simulink model "soc_dvbs2_fpga"  (R2025b)
settings: Solver=FixedStepDiscrete  StartTime=0.0  StopTime=0  RelTol=1e-3
InitFcn:
  | soc_dvbs2_init;
values from neighbouring files (symbols this model uses):
  Rsym = 4e6    (= 4000000)    [soc_dvbs2_init.m]
  soc_dvbs2_txPacketBits = [1 1 0 1 0 1 1 1 0 1 1 1 ... (2972 elements, 2972x1)]    [soc_dvbs2_txPacketBits.mat]
  syncWord = (dec2bin(hex2dec('AC')) - '0').'    [soc_dvbs2_init.m]
  txDataOut = txobj(frameBits(:))    [soc_dvbs2_init.m]
  txFiltCoeff = txobj.pTxFilterCoeff    [soc_dvbs2_init.m]
undefined symbols (not defined in the file or in its folder): Add, coefficientsLog, coefficientsSqrt1, coefficientsSqrt2, dataBits, designMultirateFIR, noisePow, NumBits1, NumBits2, seedsURNG1, seedsURNG2, Shift, Slope1, Slope2, soc_dvbs2_designFIRFilter, txDataOutS1, txDataOutS10, txDataOutS12, txDataOutS13, txDataOutS14, txDataOutS15, txDataOutS16, txDataOutS18, txDataOutS19, txDataOutS2, txDataOutS20, txDataOutS21, txDataOutS22, txDataOutS24, txDataOutS25, txDataOutS26, txDataOutS27, txDataOutS3, txDataOutS4, txDataOutS5, txDataOutS6, txDataOutS7, txDataOutS8, txDataOutS9
libraries: simulink x214, hdlsllib x211, dspsigops x22, dsphdlfiltering2 x8, dsphdlsigops2 x5, commseqgen3 x5, dsphdlmathfun2 x3, hwlogicconnlib x2, whdledac x2, commhdlcrc x2, whdlutilities x1, whdlmod x1
(part 7 of 12)

== system soc_dvbs2_fpga/DVBS2/DVBS2 TxRx/DVB-S2 HDL Receiver/Synchronizer and PL Header Decoder/Time Frequency and Coarse Phase Synchronizer/Coarse Phase Synchronizer/Coarse Phase Estimator ==
  dataIn : Inport
  pilotIdx : Inport  Port=2
  pilotValid : Inport  Port=3
  Add3 : Sum  Inputs=++|  OutDataTypeStr=Inherit: Inherit via back propagation
  Compare To Constant1 : simulink/Logic and Bit Operations/Compare To Constant  relop===  const=config.PilotMaxIdx  OutDataTypeStr=boolean
  Compare To Constant2 : simulink/Logic and Bit Operations/Compare To Constant  relop===  const=config.PilotMinIdx  OutDataTypeStr=boolean
  Data Type Duplicate : DataTypeDuplicate
  Data Type Conversion : DataTypeConversion  OutDataTypeStr=fixdt(1,17,14)  SaturateOnIntegerOverflow=off  RndMeth=Floor
  Delay{,1,15..17} (5 alike) : Delay  DelayLength=1
  Delay{8..11} (4 alike) : Delay  DelayLength=1  InitialCondition=0
  Delay{2..7,12..14,20} (10 alike) : Delay  InitialCondition=0
  Gain : Gain  Gain=conj(config.Pilot)  OutDataTypeStr=Inherit: Same as input
      mask init:
      | Simulink.suppressDiagnostic(gcb, 'SimulinkFixedPoint:util:fxpParameterPrecisionLoss');
  Gain1 : Gain  Gain=1/32  ParamDataTypeStr=fixdt(0,5,5)  OutDataTypeStr=Inherit: Same as input
  Logical Operator : Logic  AllPortsSameDT=off  OutDataTypeStr=boolean
  Logical Operator1 : Logic  AllPortsSameDT=off  OutDataTypeStr=boolean
  Unit Delay Enabled Resettable Synchronous : hdlsllib/Discrete/Unit Delay Enabled Resettable Synchronous  InitialCondition=0.0  SampleTime=-1
  estimate : Outport
  estValid : Outport  Port=2
  wires:
  Delay17/1 -> estValid/1
  Delay16/1 -> Delay13/1
  Delay15/1 -> Compare To Constant1/1
  pilotValid/1 -> Delay16/1, Delay5/1, Delay/1
  Logical Operator1/1 -> Delay12/1
  Compare To Constant1/1 -> Delay14/1
  Delay13/1 -> Logical Operator1/2
  Delay14/1 -> Logical Operator1/1
  Delay12/1 -> Delay11/1
  Delay11/1 -> Delay17/1
  Data Type Conversion/1 -> Delay8/1
  Delay10/1 -> Unit Delay Enabled Resettable Synchronous/3
  Delay9/1 -> Unit Delay Enabled Resettable Synchronous/2
  Delay8/1 -> Add3/2, Data Type Duplicate/1
  Gain1/1 -> Data Type Conversion/1
  Delay3/1 -> Delay9/1
  Delay2/1 -> Gain1/1
  Add3/1 -> Unit Delay Enabled Resettable Synchronous/1, Data Type Duplicate/2
  Delay20/1 -> Delay10/1
  Unit Delay Enabled Resettable Synchronous/1 -> Add3/1, estimate/1
  Delay7/1 -> Delay3/1
  Delay6/1 -> Logical Operator/1
  Delay5/1 -> Logical Operator/2
  Delay4/1 -> Gain/1
  Compare To Constant2/1 -> Delay6/1
  Logical Operator/1 -> Delay20/1
  Delay1/1 -> Delay4/1
  Gain/1 -> Delay2/1
  pilotIdx/1 -> Delay15/1, Compare To Constant2/1
  Delay/1 -> Delay7/1
  dataIn/1 -> Delay1/1

== system soc_dvbs2_fpga/DVBS2/DVBS2 TxRx/DVB-S2 HDL Receiver/Synchronizer and PL Header Decoder/Time Frequency and Coarse Phase Synchronizer/Coarse Phase Synchronizer/Unwrapping algorithm ==
  note: Wrap on overflow with data type
      | signed and 1 intergral bit
      | will wrap the output to
      | lie in between -1 to 1
  u : Inport
  E : Inport  Port=2
  Add : Sum  Inputs=+-  OutDataTypeStr=Inherit: Same as first input
  Add1 : Sum  Inputs=|++  OutDataTypeStr=Inherit: Same as first input
  Complex to Magnitude-Angle HDL Optimized : dsphdlmathfun2/Complex to Magnitude-Angle  NumIterationsSource=Auto  NumIterations=10  OutputFormat=Angle  AngleFormat=Normalized  ScaleOutput=on  ScalingMethod=Shift-Add  SimulateUsing=Code generation
  Constant : Constant  Value=true  SampleTime=-1
  Data Type Conversion : DataTypeConversion  OutDataTypeStr=fixdt(1,25,20)  SaturateOnIntegerOverflow=off  RndMeth=Floor
  Data Type Conversion1 : DataTypeConversion  OutDataTypeStr=fixdt(1,21,21)  SaturateOnIntegerOverflow=off  RndMeth=Floor
  Data Type Conversion2 : DataTypeConversion  OutDataTypeStr=fixdt(1,21,0)  ConvertRealWorld=Stored Integer (SI)  SaturateOnIntegerOverflow=off  RndMeth=Floor
  Gain1 : Gain  Gain=1/2  ParamDataTypeStr=fixdt(0,1,1)
  NCO HDL Optimized : dsphdlsigops2/NCO  PhaseIncrementSource=Property  PhaseIncrement=0  PhaseOffsetSource=Input port  PhaseOffset=0  DitherSource=None  NumDitherBits=4  SamplesPerFrame=1  LUTCompress=off  ResetAction=off  Waveform=Complex exponential  PhasePort=off  SimulateUsing=Code generation  AccumulatorWL=21  PhaseQuantization=on  NumQuantizerAccumulatorBits=14  OutputDataType=Binary point scaling  OutputWL=16  OutputFL=14
  PrevEst : hdlsllib/Discrete/Unit Delay Enabled Synchronous  InitialCondition=0.0  SampleTime=-1
  Terminator : Terminator
  currentEst : hdlsllib/Discrete/Unit Delay Enabled Synchronous  InitialCondition=0.0  SampleTime=-1
  estimate : Outport  VectorParamsAs1DForOutWhenUnconnected=off
  wires:
  Add/1 -> Data Type Conversion/1
  PrevEst/1 -> Add1/2, Add/2
  NCO HDL Optimized/2 -> Terminator/1
  Constant/1 -> NCO HDL Optimized/2
  Data Type Conversion2/1 -> NCO HDL Optimized/1
  Data Type Conversion1/1 -> Data Type Conversion2/1
  Data Type Conversion/1 -> Add1/1
  Complex to Magnitude-Angle HDL Optimized/1 -> currentEst/1
  E/1 -> Complex to Magnitude-Angle HDL Optimized/2
  Gain1/1 -> Data Type Conversion1/1
  NCO HDL Optimized/1 -> estimate/1
  Add1/1 -> PrevEst/1, Gain1/1
  currentEst/1 -> Add/1
  Complex to Magnitude-Angle HDL Optimized/2 -> currentEst/2, PrevEst/2
  u/1 -> Complex to Magnitude-Angle HDL Optimized/1

== system soc_dvbs2_fpga/DVBS2/DVBS2 TxRx/DVB-S2 HDL Receiver/Synchronizer and PL Header Decoder/Time Frequency and Coarse Phase Synchronizer/Fine Frequency Synchronizer/Modified L and R Algorithm ==
  z : Inport
  zvalid : Inport  Port=2
  pilotIdx : Inport  Port=3
  Compare To Constant2 : simulink/Logic and Bit Operations/Compare To Constant  relop===  const=config.PilotMaxIdx  OutDataTypeStr=boolean
  Complex to Magnitude-Angle HDL Optimized : dsphdlmathfun2/Complex to Magnitude-Angle  NumIterationsSource=Auto  NumIterations=10  OutputFormat=Angle  AngleFormat=Normalized  ScaleOutput=on  ScalingMethod=Shift-Add  SimulateUsing=Code generation
  Data Type Conversion : DataTypeConversion  OutDataTypeStr=fixdt(1,21,21)  SaturateOnIntegerOverflow=off  RndMeth=Floor
  Data Type Conversion1 : DataTypeConversion  OutDataTypeStr=fixdt(1,43,26)  SaturateOnIntegerOverflow=off  RndMeth=Floor
  Data Type Conversion3 : DataTypeConversion  OutDataTypeStr=fixdt(1,43,40)  ConvertRealWorld=Stored Integer (SI)  SaturateOnIntegerOverflow=off  RndMeth=Floor
  Delay : Delay
  Delay1 : Delay
  Delay2 : Delay
  Delay3 : Delay  DelayLength=28
  Delay4 : Delay  DelayLength=1
  Gain : Gain  Gain=fi(1/19,0,16,16)  ParamDataTypeStr=Inherit: Inherit from 'Gain'  OutDataTypeStr=Inherit: Same as input
  L and R Algorithm 18 point : Subsystem
  Logical Operator : Logic  AllPortsSameDT=off  OutDataTypeStr=boolean
  Moving Average : Subsystem
  Terminator : Terminator
  Unit Delay Enabled Synchronous : hdlsllib/Discrete/Unit Delay Enabled Synchronous  InitialCondition=0.0  SampleTime=-1
  estOut : Outport
  wires:
  Complex to Magnitude-Angle HDL Optimized/2 -> Terminator/1, Unit Delay Enabled Synchronous/2
  Unit Delay Enabled Synchronous/1 -> Delay4/1
  Data Type Conversion1/1 -> Data Type Conversion3/1
  Moving Average/2(validOut) -> Complex to Magnitude-Angle HDL Optimized/2
  Data Type Conversion3/1 -> Complex to Magnitude-Angle HDL Optimized/1
  Complex to Magnitude-Angle HDL Optimized/1 -> Unit Delay Enabled Synchronous/1
  z/1 -> L and R Algorithm 18 point/1(z)
  Moving Average/1(dataOut) -> Data Type Conversion1/1
  Logical Operator/1 -> Delay3/1
  Compare To Constant2/1 -> Logical Operator/2
  Delay4/1 -> Delay1/1
  Delay2/1 -> Data Type Conversion/1
  Delay1/1 -> Gain/1
  Delay3/1 -> Delay/1
  Data Type Conversion/1 -> estOut/1
  Gain/1 -> Delay2/1
  zvalid/1 -> L and R Algorithm 18 point/2(zvalid), Logical Operator/1
  L and R Algorithm 18 point/1(dataIn) -> Moving Average/1(dataIn)
  Delay/1 -> Moving Average/2(validIn)
  pilotIdx/1 -> Compare To Constant2/1

== system soc_dvbs2_fpga/DVBS2/DVBS2 TxRx/DVB-S2 HDL Receiver/Synchronizer and PL Header Decoder/Time Frequency and Coarse Phase Synchronizer/Fine Gain Control/Reciprocal ==
  dataIn : Inport
  Compare To Constant : simulink/Logic and Bit Operations/Compare To Constant  relop=<  const=0  OutDataTypeStr=boolean
  Compare To Constant1 : simulink/Logic and Bit Operations/Compare To Constant  relop===  const=0  OutDataTypeStr=boolean
  Constant : Constant  OutDataTypeStr=Inherit: Inherit via back propagation  SampleTime=-1
  Data Type Duplicate : DataTypeDuplicate
  Data Type Conversion : DataTypeConversion  OutDataTypeStr=fixdt(1,WL,0)  ConvertRealWorld=Stored Integer (SI)  SaturateOnIntegerOverflow=off  RndMeth=Floor
  Data Type Conversion1 : DataTypeConversion  OutDataTypeStr=fixdt(0,LUTAddrWL,0)  ConvertRealWorld=Stored Integer (SI)  SaturateOnIntegerOverflow=off  RndMeth=Floor
      mask init:
      | Simulink.suppressDiagnostic(gcb, 'SimulinkFixedPoint:util:Overflowoccurred');
  Data Type Conversion2 : DataTypeConversion  OutDataTypeStr=fixdt(0,WL-LUTAddrWL,0)  ConvertRealWorld=Stored Integer (SI)  SaturateOnIntegerOverflow=off  RndMeth=Floor
  Delay : Delay  DelayLength=1
  Delay1 : Delay  DelayLength=1
  Delay2 : Delay  DelayLength=1
  Delay3 : Delay  DelayLength=7
  Extract Bits : simulink/Logic and Bit Operations/Extract Bits  bitsToExtract=Range ending with least significant bit  numBits=LUTAddrWL  bitIdxRange=[0 7]  outScalingMode=Treat bit field as an integer
  Function Impl : Subsystem
  Switch : Switch  Criteria=u2 > Threshold  SaturateOnIntegerOverflow=off  InputSameDT=off
  dataOut : Outport
  wires:
  Constant/1 -> Switch/1, Data Type Duplicate/1
  Compare To Constant1/1 -> Switch/2
  Delay3/1 -> Compare To Constant1/1
  Switch/1 -> dataOut/1
  Data Type Conversion2/1 -> Function Impl/1(switch)
  Delay2/1 -> Data Type Conversion1/1
  Delay1/1 -> Data Type Conversion2/1
  Delay/1 -> Extract Bits/1, Compare To Constant/1
  Function Impl/1(functionValues) -> Switch/3, Data Type Duplicate/2
  Data Type Conversion1/1 -> Function Impl/2(LUTAddr)
  Compare To Constant/1 -> Delay1/1
  Data Type Conversion/1 -> Delay/1
  Extract Bits/1 -> Delay2/1
  dataIn/1 -> Data Type Conversion/1, Delay3/1

== system soc_dvbs2_fpga/DVBS2/DVBS2 TxRx/DVB-S2 HDL Receiver/Synchronizer and PL Header Decoder/Time Frequency and Coarse Phase Synchronizer/Time and Coarse Frequency Synchronizer/Coarse Frequency Estimator ==
  rst : Inport
  dataIn : Inport  Port=2
  pilotValid : Inport  Port=3
  pilotIdx : Inport  Port=4
  Compare To Constant : simulink/Logic and Bit Operations/Compare To Constant  relop=>  const=32  OutDataTypeStr=boolean
  Constant : Constant  Value=CFCV  OutDataTypeStr=boolean  SampleTime=-1
  Delay : Delay  DelayLength=1  InitialCondition=1
  Delay{1..4,28} (5 alike) : Delay  DelayLength=1
  Direct Digital Synthesis : Subsystem
  Frequency Error Detector : Subsystem
  Logical Operator : Logic  Operator=NOT  AllPortsSameDT=off  OutDataTypeStr=boolean
  Loop Filter : Subsystem
  Multiport Switch : MultiPortSwitch  DataPortOrder=Zero-based contiguous  Inputs=2  zeroidx=on  SaturateOnIntegerOverflow=off  InputSameDT=off
  Pilot Blks Counter : Subsystem
  Unit Delay Enabled Resettable Synchronous : hdlsllib/Discrete/Unit Delay Enabled Resettable Synchronous  InitialCondition=0  SampleTime=-1
  complexEstimate : Outport
  normFreqEst : Outport  Port=2
  wires:
  Loop Filter/2(rstOut) -> Delay4/1
  Delay4/1 -> Direct Digital Synthesis/2(rst)
  Logical Operator/1 -> Delay1/1
  rst/1 -> Pilot Blks Counter/3(rst), Unit Delay Enabled Resettable Synchronous/3, Delay2/1
  Unit Delay Enabled Resettable Synchronous/1 -> Logical Operator/1
  pilotValid/1 -> Pilot Blks Counter/2(pilotValid), Frequency Error Detector/3(pilotValid)
  Pilot Blks Counter/1(pilotBlkCount) -> Compare To Constant/1
  pilotIdx/1 -> Pilot Blks Counter/1(pilotIdx), Frequency Error Detector/2(pilotIdx)
  Compare To Constant/1 -> Unit Delay Enabled Resettable Synchronous/2, Unit Delay Enabled Resettable Synchronous/1
  Delay3/1 -> Direct Digital Synthesis/1(v)
  Delay2/1 -> Loop Filter/2(rst)
  Delay1/1 -> Loop Filter/3(En)
  Delay28/1 -> Loop Filter/1(e)
  Loop Filter/1(v) -> Delay3/1
  Direct Digital Synthesis/2(normalizedEst) -> normFreqEst/1
  Direct Digital Synthesis/1(complexEst) -> Multiport Switch/3
  dataIn/1 -> Frequency Error Detector/1(dataIn)
  Delay/1 -> Multiport Switch/2
  Constant/1 -> Multiport Switch/1
  Multiport Switch/1 -> complexEstimate/1, Delay/1
  Frequency Error Detector/1(e) -> Delay28/1

== system soc_dvbs2_fpga/DVBS2/DVBS2 TxRx/DVB-S2 HDL Receiver/Synchronizer and PL Header Decoder/Time Frequency and Coarse Phase Synchronizer/Time and Coarse Frequency Synchronizer/Frame Synchronizer ==
  dataIn : Inport
  validIn : Inport  Port=2
  Correlator : Subsystem
  Data Type Conversion : DataTypeConversion  OutDataTypeStr=fixdt(1,15,12)  SaturateOnIntegerOverflow=off  RndMeth=Floor
  Data Type Conversion1 : DataTypeConversion  OutDataTypeStr=fixdt(1,15,11)  SaturateOnIntegerOverflow=off  RndMeth=Floor
  Data Type Conversion2 : DataTypeConversion  OutDataTypeStr=fixdt(1,15,12)  SaturateOnIntegerOverflow=off  RndMeth=Floor
  Delay1 : Delay  DelayLength=70
  Delay{6,9..11} (4 alike) : Delay  DelayLength=9
  Delay12 : Delay
  Delay13 : Delay
  Delay2 : Delay  DelayLength=70
  Delay3 : Delay  DelayLength=config.PLSCLength
  Delay4 : Delay  DelayLength=config.PLSCLength
  Delay5 : Delay  DelayLength=config.PLSCLength
  Pilot and Sync Pulse Indicator : Subsystem
      settings: PortSchema="{\"entries\":[{\"content\":{\"sides\":[{\"content\":{\"connectorIds\":[\"In1\",\"In2\",\"In3\"]},\"type\":\"ConnectorPlacement.EquallySpacedRectSide\",\"uuid\":\"f5659eee-e56d-4f51-b3c8-0bb5849d1c90\"},{\"content\":{\"connectorIds\":[\"Out1\",\"Out2\"],\"side\":\"RIGHT\"},\"type\":\"ConnectorPlacement.EquallySpacedRectSide\",\"uuid\":\"967999ef-0aaf-4de1-9521-cd04737cc7dc\"},{\"content\":{\"connectorIds\":[\"Out3\"],\"side\":\"TOP\"},\"type\":\"ConnectorPlacement.EquallySpacedRectSide\",\"uuid\":\"20532451-5348-4d64-b061-3cd12226f9ee\"}]},\"type\":\"ConnectorPlacement.EquallySpacedConnector\",\"uuid\":\"2e00dd47-a2f7-4f59-b412-aa328ab3c5d1\"}],\"packageUris\":[\"http://schema.mathworks.com/mf0/Connector/R2020b\"],\"version\":\"1.0\"}"
  dataOut : Outport
  validOut : Outport  Port=2
  endOfSOF : Outport  Port=3
  hasPilots : Outport  Port=4
  VisualizeCorrelationSignals : Outport  Port=5
  wires:
  Data Type Conversion2/1 -> Pilot and Sync Pulse Indicator/3(threshold)
  Data Type Conversion1/1 -> Pilot and Sync Pulse Indicator/2(PLSCCorr)
  Data Type Conversion/1 -> Pilot and Sync Pulse Indicator/1(SOFCorrDelayed)
  Pilot and Sync Pulse Indicator/1(hasPilots) -> hasPilots/1
  Delay9/1 -> validOut/1
  Pilot and Sync Pulse Indicator/2(thresholdExceeded) -> endOfSOF/1
  Delay10/1 -> dataOut/1
  Correlator/1(SOFCorrOut) -> Delay5/1
  Correlator/3(threshold) -> Data Type Conversion2/1
  Correlator/2(PLSCCorrOut) -> Data Type Conversion1/1
  Delay12/1 -> Delay6/1, Correlator/1(dataIn)
  dataIn/1 -> Delay12/1
  validIn/1 -> Delay13/1
  Delay6/1 -> Delay1/1
  Delay11/1 -> Delay2/1
  Delay4/1 -> Delay9/1
  Delay3/1 -> Delay10/1
  Delay5/1 -> Data Type Conversion/1
  Delay2/1 -> Delay4/1
  Delay1/1 -> Delay3/1
  Delay13/1 -> Delay11/1, Correlator/2(validIn)
  Pilot and Sync Pulse Indicator/3(VisualizeCorrelationSignals) -> VisualizeCorrelationSignals/1

== system soc_dvbs2_fpga/DVBS2/DVBS2 TxRx/DVB-S2 HDL Receiver/Synchronizer and PL Header Decoder/Time Frequency and Coarse Phase Synchronizer/Time and Coarse Frequency Synchronizer/PL Data Descrambler and Pilot Valid Indicator ==
  dataIn : Inport
  validIn : Inport  Port=2
  endOfSOFIn : Inport  Port=3
  hasPilots : Inport  Port=4
  Compare To Constant1 : simulink/Logic and Bit Operations/Compare To Constant  relop===  const=config.PLSCLength - 1  OutDataTypeStr=boolean
  Delay : Delay  DelayLength=config.SOFLength
  Delay1 : Delay  DelayLength=config.SOFLength
  Delay{2..18} (17 alike) : Delay  DelayLength=1
  Delay{19..22} (4 alike) : Delay  DelayLength=14
  Delay23 : Delay  DelayLength=4
  Delay24 : Delay  DelayLength=4
  Input Sample Counter : hdlsllib/Sources/HDL Counter  CountType=Free running  CountInit=0  CountStep=1  CountMax=25  CountFromType=Initial value  CountFrom=0  CountResetPort=on  CountLoadPort=off  CountEnbPort=on  CountDirPort=off  CountHitOutputPort=off  CountDataType=Unsigned  CountWordLen=32  CountFracLen=0  CountSampTime=1
  Logical Operator : Logic  AllPortsSameDT=off  OutDataTypeStr=boolean
  PL Data Descrambler : Subsystem
  Pilot Valid Indicator : Subsystem
  pilotidx : Outport
  pilotValid : Outport  Port=2
  dataOut : Outport  Port=3
  validOut : Outport  Port=4
  endOfSOF : Outport  Port=5
  wires:
  Delay10/1 -> Delay8/1
  dataIn/1 -> Delay10/1
  Delay24/1 -> validOut/1
  Delay23/1 -> dataOut/1
  Delay22/1 -> Pilot Valid Indicator/1(pilotEnable)
  Delay21/1 -> Pilot Valid Indicator/2(validIn)
  Delay20/1 -> Pilot Valid Indicator/3(endOfSOFIn)
  Delay19/1 -> Pilot Valid Indicator/4(endOfPLSC)
  Delay18/1 -> Delay22/1
  Delay17/1 -> Delay21/1
  Delay16/1 -> Delay20/1
  Delay15/1 -> Logical Operator/1
  Delay14/1 -> Logical Operator/2
  Delay13/1 -> PL Data Descrambler/2(inputCount)
  Delay12/1 -> PL Data Descrambler/3(validIn)
  Delay11/1 -> PL Data Descrambler/4(dataIn)
  Delay8/1 -> Delay11/1
  Delay7/1 -> Delay12/1, [validIn]
  Delay6/1 -> Delay13/1, Compare To Constant1/1
  Delay5/1 -> Delay16/1
  Delay4/1 -> Delay18/1
  Delay3/1 -> Delay4/1
  Delay2/1 -> Input Sample Counter/1, Delay5/1
  Delay9/1 -> Input Sample Counter/2, Delay7/1
  Logical Operator/1 -> PL Data Descrambler/1(reset), Delay19/1
  Pilot Valid Indicator/3(endOfSOF) -> endOfSOF/1
  Pilot Valid Indicator/2(pilotIdx) -> pilotidx/1
  Pilot Valid Indicator/1(pilotValid) -> pilotValid/1
  Delay1/1 -> Delay24/1
  Delay/1 -> Delay23/1
  PL Data Descrambler/2(validOut) -> Delay1/1
  PL Data Descrambler/1(dataOut) -> Delay/1
  validIn/1 -> Delay9/1
  [validIn] -> Delay17/1
  [validIn] -> Delay15/1
  hasPilots/1 -> Delay3/1
  endOfSOFIn/1 -> Delay2/1
  Compare To Constant1/1 -> Delay14/1
  Input Sample Counter/1 -> Delay6/1

== system soc_dvbs2_fpga/DVBS2/DVBS2 TxRx/DVB-S2 HDL Receiver/Synchronizer and PL Header Decoder/Time Frequency and Coarse Phase Synchronizer/Time and Coarse Frequency Synchronizer/Symbol Synchronizer ==
  dataIn : Inport
  validIn : Inport  Port=2
  Data Type Duplicate : DataTypeDuplicate
  Data Type Conversion : DataTypeConversion  SaturateOnIntegerOverflow=off  RndMeth=Floor
  Delay{1..4,6,8..9} (7 alike) : Delay  DelayLength=1
  Delay5 : Delay  DelayLength=12
  Delay7 : Delay  DelayLength=12
  Gardner TED : Subsystem
  Integer Delay{1..4} (4 alike) : Delay  DelayLength=1
  Interpolation Control : MATLAB Function
  Interpolation Filter : Subsystem
  Loop Filter : Subsystem
  Rate Handle : Subsystem
  dataOut : Outport
  validOut : Outport  Port=2
  wires:
  Delay9/1 -> Gardner TED/2(strobe)
  Delay8/1 -> Gardner TED/1(data)
  Integer Delay2/1 -> Delay7/1
  Integer Delay1/1 -> Interpolation Filter/1(In)
  Delay5/1 -> Delay2/1, Delay9/1
  Delay2/1 -> Rate Handle/2(strobe)
  Rate Handle/1(dataOut) -> dataOut/1
  Rate Handle/2(validOut) -> validOut/1
  validIn/1 -> Integer Delay2/1
  Delay7/1 -> Delay6/1
  Delay6/1 -> Rate Handle/3(validIn)
  Delay4/1 -> Interpolation Control/1(Delta)
  Delay3/1 -> Loop Filter/1(e)
  Integer Delay3/1 -> Delay5/1
  Interpolation Control/2(Underflow) -> Integer Delay3/1
  Gardner TED/1(e) -> Delay3/1
  Loop Filter/1(v) -> Delay4/1
  Interpolation Filter/1(interpolant) -> Data Type Conversion/1, Delay8/1
  Delay1/1 -> Rate Handle/1(dataIn)
  Data Type Conversion/1 -> Data Type Duplicate/2, Delay1/1
  Integer Delay4/1 -> Interpolation Filter/2(mu)
  dataIn/1 -> Integer Delay1/1, Data Type Duplicate/1
  Interpolation Control/1(mu) -> Integer Delay4/1

== system soc_dvbs2_fpga/DVBS2/DVBS2 TxRx/DVB-S2 HDL Receiver/Synchronizer and PL Header Decoder/Time Frequency and Coarse Phase Synchronizer/Variance Estimator/Moving Average  ==
  enable : Inport
  dataIn : Inport  Port=2
  Add1 : Sum  Inputs=|+-  OutDataTypeStr=Inherit: Same as first input
  Add2 : Sum  Inputs=|++  OutDataTypeStr=Inherit: Same as first input
  Data Type Conversion : DataTypeConversion  OutDataTypeStr=fixdt(1,32,30)  SaturateOnIntegerOverflow=off  RndMeth=Floor
  Delay : Delay  DelayLength=2048  ShowEnablePort=on
      settings: InputPortMap=u0,e6
  Delay1 : Delay  DelayLength=1  ShowEnablePort=on
      settings: InputPortMap=u0,e6
  Delay{2,4..5,22} (4 alike) : Delay
  Delay3 : Delay  DelayLength=1  ShowEnablePort=on
      settings: InputPortMap=u0,e6
  Gain : Gain  Gain=1/2048  ParamDataTypeStr=fixdt(0,11,11)
  avgOut : Outport  InitialOutput=0
  wires:
  Data Type Conversion/1 -> Delay2/1
  Delay2/1 -> Add2/1
  Delay22/1 -> Gain/1
  dataIn/1 -> Delay/1, Add1/1
  Gain/1 -> Data Type Conversion/1
  Delay/1 -> Add1/2
  Add2/1 -> Delay3/1, Delay1/1
  Add1/1 -> Delay22/1
  Delay1/1 -> Add2/2
  Delay3/1 -> avgOut/1
  enable/1 -> Delay4/1, Delay/2
  Delay4/1 -> Delay5/1
  Delay5/1 -> Delay1/2, Delay3/2

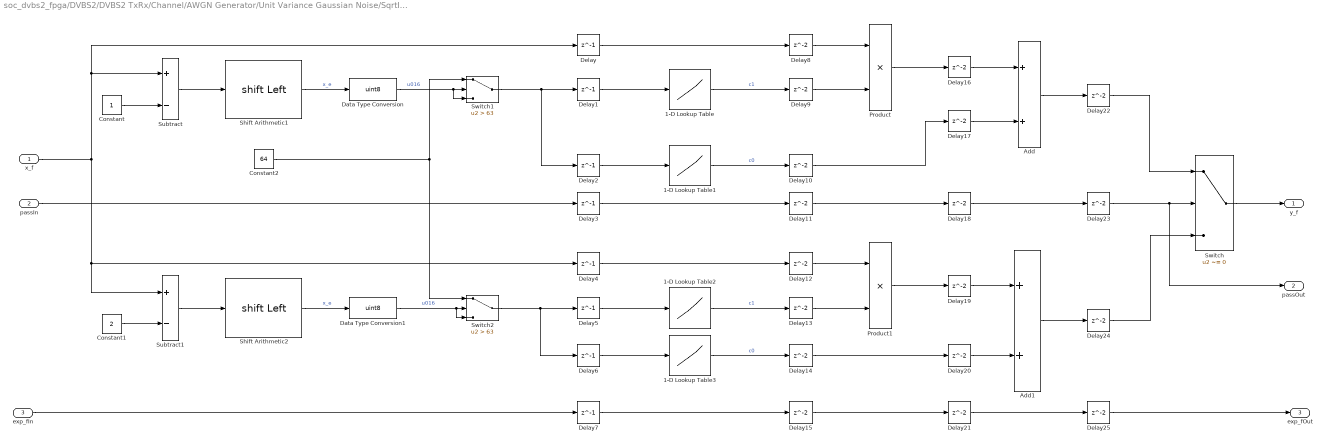
== system soc_dvbs2_fpga/DVBS2/DVBS2 TxRx/Channel/AWGN Generator/Unit Variance Gaussian Noise/SqrtImplementation/SqrtEval/FunctionEvaluation ==
  x_f : Inport
  passIn : Inport  Port=2
  exp_fIn : Inport  Port=3
  1-D Lookup Table : Lookup_n-D  NumberOfTableDimensions=1  LookupTableObject=''  BreakpointsForDimension1=[0:64]  BreakpointsForDimension1FirstPoint=10  BreakpointsForDimension2FirstPoint=10  BreakpointsForDimension1Spacing=12  BreakpointsForDimension2Spacing=12  IndexSearchMethod=Evenly spaced points  Table=[coefficientsSqrt1(:,1)' 0]  InterpMethod=Flat  DiagnosticForOutOfRangeInput=Error  InternalRulePriority=Speed  OutDataTypeStr=fixdt(1,13,12)  RndMeth=Simplest
  1-D Lookup Table1 : Lookup_n-D  NumberOfTableDimensions=1  LookupTableObject=''  BreakpointsForDimension1=0:64  BreakpointsForDimension1FirstPoint=10  BreakpointsForDimension2FirstPoint=10  BreakpointsForDimension1Spacing=12  BreakpointsForDimension2Spacing=12  IndexSearchMethod=Evenly spaced points  Table=[coefficientsSqrt1(:,2)' 0]  InterpMethod=Flat  DiagnosticForOutOfRangeInput=Error  InternalRulePriority=Speed  OutDataTypeStr=fixdt(1,21,20)  RndMeth=Simplest
  1-D Lookup Table2 : Lookup_n-D  NumberOfTableDimensions=1  LookupTableObject=''  BreakpointsForDimension1=0:64  BreakpointsForDimension1FirstPoint=10  BreakpointsForDimension2FirstPoint=10  BreakpointsForDimension1Spacing=12  BreakpointsForDimension2Spacing=12  IndexSearchMethod=Evenly spaced points  Table=[coefficientsSqrt2(:,1)' 0]  InterpMethod=Flat  DiagnosticForOutOfRangeInput=Error  InternalRulePriority=Speed  OutDataTypeStr=fixdt(1,13,12)  RndMeth=Simplest
  1-D Lookup Table3 : Lookup_n-D  NumberOfTableDimensions=1  LookupTableObject=''  BreakpointsForDimension1=0:64  BreakpointsForDimension1FirstPoint=10  BreakpointsForDimension2FirstPoint=10  BreakpointsForDimension1Spacing=12  BreakpointsForDimension2Spacing=12  IndexSearchMethod=Evenly spaced points  Table=[coefficientsSqrt2(:,2)' 0]  InterpMethod=Flat  DiagnosticForOutOfRangeInput=Error  InternalRulePriority=Speed  OutDataTypeStr=fixdt(1,21,20)  RndMeth=Simplest
  Add : Sum  OutDataTypeStr=fixdt(0,17,13)
  Add1 : Sum  AccumDataTypeStr=fixdt(0,17,13)
  Constant : Constant  OutDataTypeStr=uint8  SampleTime=-1
  Constant1 : Constant  Value=2  OutDataTypeStr=uint8  SampleTime=-1
  Constant2 : Constant  Value=64  OutDataTypeStr=uint8  SampleTime=-1
  Data Type Conversion : DataTypeConversion  OutDataTypeStr=uint8  SaturateOnIntegerOverflow=off  RndMeth=Floor
  Data Type Conversion1 : DataTypeConversion  OutDataTypeStr=uint8  SaturateOnIntegerOverflow=off  RndMeth=Floor
  Delay{,1..7} (8 alike) : Delay  DelayLength=1
  Delay{8..25} (18 alike) : Delay
  Product : Product
  Product1 : Product
  Shift Arithmetic1 : ArithShift  BinPtShiftNumber=6  BitShiftDirection=Left
  Shift Arithmetic2 : ArithShift  BinPtShiftNumber=5  BitShiftDirection=Left
  Subtract : Sum  Inputs=+-
  Subtract1 : Sum  Inputs=+-  AccumDataTypeStr=fixdt(0,31,24)
  Switch : Switch  Criteria=u2 ~= 0  SaturateOnIntegerOverflow=off  InputSameDT=off
  Switch1 : Switch  Criteria=u2 > Threshold  Threshold=63  SaturateOnIntegerOverflow=off  InputSameDT=off
  Switch2 : Switch  Criteria=u2 > Threshold  Threshold=63  OutDataTypeStr=int8  SaturateOnIntegerOverflow=off  InputSameDT=off
  y_f : Outport
  passOut : Outport  Port=2
  exp_fOut : Outport  Port=3
  wires:
  1-D Lookup Table1/1 -> Delay10/1  "c0"
  Switch/1 -> y_f/1
  Shift Arithmetic2/1 -> Data Type Conversion1/1  "x_e"
  1-D Lookup Table2/1 -> Delay13/1  "c1"
  1-D Lookup Table3/1 -> Delay14/1  "c0"
  Shift Arithmetic1/1 -> Data Type Conversion/1  "x_e"
  1-D Lookup Table/1 -> Delay9/1  "c1"
  Add/1 -> Delay22/1
  Add1/1 -> Delay24/1
  Constant/1 -> Subtract/2
  Constant1/1 -> Subtract1/2
  Constant2/1 -> Switch2/1, Switch1/1
  Data Type Conversion/1 -> Switch1/2, Switch1/3  "u016"
  Data Type Conversion1/1 -> Switch2/3, Switch2/2  "u016"
  Subtract/1 -> Shift Arithmetic1/1
  Subtract1/1 -> Shift Arithmetic2/1
  Switch2/1 -> Delay5/1, Delay6/1
  Switch1/1 -> Delay1/1, Delay2/1
  Product1/1 -> Delay19/1
  Product/1 -> Delay16/1
  passIn/1 -> Delay3/1
  x_f/1 -> Delay4/1, Subtract1/1, Delay/1, Subtract/1
  Delay/1 -> Delay8/1
  Delay1/1 -> 1-D Lookup Table/1
  Delay2/1 -> 1-D Lookup Table1/1
  Delay3/1 -> Delay11/1
  Delay4/1 -> Delay12/1
  Delay5/1 -> 1-D Lookup Table2/1
  Delay6/1 -> 1-D Lookup Table3/1
  exp_fIn/1 -> Delay7/1
  Delay7/1 -> Delay15/1
  Delay8/1 -> Product/1
  Delay9/1 -> Product/2
  Delay10/1 -> Delay17/1
  Delay11/1 -> Delay18/1
  Delay12/1 -> Product1/1
  Delay13/1 -> Product1/2
  Delay14/1 -> Delay20/1
  Delay15/1 -> Delay21/1
  Delay16/1 -> Add/1
  Delay17/1 -> Add/2
  Delay18/1 -> Delay23/1
  Delay19/1 -> Add1/1
  Delay20/1 -> Add1/2
  Delay21/1 -> Delay25/1
  Delay22/1 -> Switch/1
  Delay23/1 -> passOut/1, Switch/2
  Delay24/1 -> Switch/3
  Delay25/1 -> exp_fOut/1

== system soc_dvbs2_fpga/DVBS2/DVBS2 TxRx/Channel/AWGN Generator/Unit Variance Gaussian Noise/SqrtImplementation/SqrtEval/RangeReconstruction ==
  y_f : Inport
  pass : Inport  Port=2
  exp_f : Inport  Port=3
  Add : Sum  AccumDataTypeStr=int8
  Constant : Constant  OutDataTypeStr=int8  SampleTime=-1
  Delay{1..3,8} (4 alike) : Delay
  Delay{4..7,9..12} (8 alike) : Delay  DelayLength=1
  Gain : Gain  Gain=-1  OutDataTypeStr=int8
  Shift Arithmetic : ArithShift  BitShiftNumber=1
  Shift Arithmetic1 : ArithShift  BitShiftNumberSource=Input port  BitShiftNumber=8
      settings: InputPortMap=u0,p1
  Switch : Switch  Criteria=u2 ~= 0  SaturateOnIntegerOverflow=off  InputSameDT=off
  f : Outport
  wires:
  Add/1 -> Delay4/1
  exp_f/1 -> Delay10/1, Delay12/1
  pass/1 -> Delay11/1
  y_f/1 -> Delay9/1
  Switch/1 -> Shift Arithmetic/1
  Constant/1 -> Add/1
  Shift Arithmetic1/1 -> f/1
  Shift Arithmetic/1 -> Delay2/1
  Gain/1 -> Delay8/1
  Delay8/1 -> Shift Arithmetic1/2
  Delay1/1 -> Shift Arithmetic1/1
  Delay2/1 -> Gain/1
  Delay3/1 -> Delay1/1
  Delay4/1 -> Switch/1
  Delay5/1 -> Delay3/1
  Delay6/1 -> Switch/3
  Delay7/1 -> Switch/2
  Delay9/1 -> Delay5/1
  Delay10/1 -> Add/2
  Delay11/1 -> Delay7/1
  Delay12/1 -> Delay6/1

== system soc_dvbs2_fpga/DVBS2/DVBS2 TxRx/Channel/AWGN Generator/Unit Variance Gaussian Noise/SqrtImplementation/SqrtEval/RangeReduction ==
  note: Range of x_f=[1,4)
  u : Inport
  Add : Sum  Inputs=+-  OutDataTypeStr=int8
  Constant : Constant  Value=5  OutDataTypeStr=uint8  SampleTime=-1
  Data Type Conversion : DataTypeConversion  OutDataTypeStr=fixdt(0,38,31)  SaturateOnIntegerOverflow=off  RndMeth=Floor
  Delay{1..20} (20 alike) : Delay  DelayLength=1
  Shift Arithmetic : ArithShift  BitShiftNumberSource=Input port  BitShiftNumber=8
      settings: InputPortMap=u0,p1
  Shift Arithmetic1 : ArithShift  BitShiftNumber=1  BitShiftDirection=Right
  Shift Arithmetic2 : ArithShift  BitShiftNumber=6  BitShiftDirection=Right
  Shift Arithmetic3 : ArithShift  BitShiftNumber=1  BitShiftDirection=Right
  Shift Arithmetic4 : ArithShift  BitShiftNumber=1  BitShiftDirection=Left
  Subtract : Sum  Inputs=+-
  Switch : Switch  Criteria=u2 ~= 0  SaturateOnIntegerOverflow=off  InputSameDT=off
  leadingZeroDetector : MATLAB Function  TreatAsAtomicUnit=on
  x_f : Outport
  pass : Outport  Port=2
  exp_f : Outport  Port=3  VectorParamsAs1DForOutWhenUnconnected=off
  wires:
  Delay2/1 -> Delay19/1
  Delay4/1 -> Add/2
  Shift Arithmetic1/1 -> Delay1/1
  Constant/1 -> Add/1
  Shift Arithmetic4/1 -> Delay9/1
  Switch/1 -> x_f/1
  Shift Arithmetic3/1 -> Delay16/1
  leadingZeroDetector/1(exp_f) -> Delay4/1
  u/1 -> Data Type Conversion/1, Delay3/1
  Shift Arithmetic/1 -> Delay11/1, Delay12/1  "x_f1"
  Add/1 -> Delay18/1
  Subtract/1 -> Delay6/1
  Data Type Conversion/1 -> Shift Arithmetic2/1
  Shift Arithmetic2/1 -> Delay20/1
  Delay1/1 -> Switch/1
  Delay5/1 -> Switch/3
  Delay6/1 -> Switch/2, pass/1
  Delay7/1 -> exp_f/1
  Delay8/1 -> Subtract/1
  Delay9/1 -> Subtract/2
  Delay10/1 -> Delay7/1
  Delay11/1 -> Delay5/1
  Delay12/1 -> Shift Arithmetic1/1
  Delay13/1 -> Shift Arithmetic/1
  Delay14/1 -> Shift Arithmetic/2
  Delay15/1 -> Delay8/1
  Delay16/1 -> Shift Arithmetic4/1
  Delay17/1 -> Delay10/1
  Delay18/1 -> Delay17/1, Delay15/1, Delay14/1, Shift Arithmetic3/1
  Delay19/1 -> Delay13/1
  Delay20/1 -> leadingZeroDetector/1(x)
  Delay3/1 -> Delay2/1

== system soc_dvbs2_fpga/DVBS2/DVBS2 TxRx/Channel/AWGN Generator/Unit Variance Gaussian Noise/logImplementation/log/FunctionEvaluation ==
  x_e : Inport
  exp_eIn : Inport  Port=2
  1-D Lookup Table : Lookup_n-D  NumberOfTableDimensions=1  LookupTableObject=''  BreakpointsForDimension1=0:255  BreakpointsForDimension1FirstPoint=10  BreakpointsForDimension2FirstPoint=10  BreakpointsForDimension1Spacing=12  BreakpointsForDimension2Spacing=12  IndexSearchMethod=Evenly spaced points  Table=coefficientsLog(:,1)  InterpMethod=Flat  DiagnosticForOutOfRangeInput=Error  InternalRulePriority=Speed  OutDataTypeStr=fixdt(1,16,15)  RndMeth=Simplest
  1-D Lookup Table1 : Lookup_n-D  NumberOfTableDimensions=1  LookupTableObject=''  BreakpointsForDimension1=0:255  BreakpointsForDimension1FirstPoint=10  BreakpointsForDimension2FirstPoint=10  BreakpointsForDimension1Spacing=12  BreakpointsForDimension2Spacing=12  IndexSearchMethod=Evenly spaced points  Table=coefficientsLog(:,2)  InterpMethod=Flat  DiagnosticForOutOfRangeInput=Error  InternalRulePriority=Speed  OutDataTypeStr=fixdt(1,16,14)  RndMeth=Simplest
  1-D Lookup Table2 : Lookup_n-D  NumberOfTableDimensions=1  LookupTableObject=''  BreakpointsForDimension1=0:255  BreakpointsForDimension1FirstPoint=10  BreakpointsForDimension2FirstPoint=10  BreakpointsForDimension1Spacing=12  BreakpointsForDimension2Spacing=12  IndexSearchMethod=Evenly spaced points  Table=coefficientsLog(:,3)  InterpMethod=Flat  DiagnosticForOutOfRangeInput=Error  InternalRulePriority=Speed  OutDataTypeStr=fixdt(1,32,30)  RndMeth=Simplest
  Add : Sum  OutDataTypeStr=fixdt(1,16,14)
  Add1 : Sum  OutDataTypeStr=fixdt(1,31,27)
  Data Type Conversion : DataTypeConversion  OutDataTypeStr=uint8  SaturateOnIntegerOverflow=off  RndMeth=Floor
  Data Type Conversion1 : DataTypeConversion  OutDataTypeStr=fixdt(0,16,15)  SaturateOnIntegerOverflow=off  RndMeth=Floor
  Delay1 : Delay  DelayLength=1
  Delay{3..30} (28 alike) : Delay
  Delay2 : Delay  DelayLength=1
  Product : Product  OutDataTypeStr=fixdt(1,16,15)
  Product1 : Product  OutDataTypeStr=fixdt(1,31,27)
  Shift Arithmetic1 : ArithShift  BinPtShiftNumber=8  BitShiftDirection=Left
  y_e : Outport
  exp_eOut : Outport  Port=2
  wires:
  Shift Arithmetic1/1 -> Data Type Conversion/1  "x_e"
  x_e/1 -> Data Type Conversion1/1, Shift Arithmetic1/1
  1-D Lookup Table/1 -> Delay22/1  "c2"
  Add1/1 -> Delay1/1
  1-D Lookup Table1/1 -> Delay25/1  "c1"
  1-D Lookup Table2/1 -> Delay26/1  "c0"
  Product/1 -> Delay10/1
  Product1/1 -> Delay3/1
  Data Type Conversion1/1 -> Delay23/1
  Add/1 -> Delay7/1
  exp_eIn/1 -> Delay30/1
  Delay3/1 -> Add1/1
  Delay1/1 -> y_e/1
  Delay2/1 -> exp_eOut/1
  Delay4/1 -> Add1/2
  Delay5/1 -> Delay2/1
  Delay6/1 -> Product1/1
  Delay7/1 -> Product1/2
  Delay8/1 -> Delay4/1
  Delay9/1 -> Delay5/1
  Delay10/1 -> Add/1
  Delay11/1 -> Delay6/1
  Delay12/1 -> Add/2
  Delay13/1 -> Delay8/1
  Delay14/1 -> Delay9/1
  Delay15/1 -> Product/1
  Delay16/1 -> Product/2
  Delay17/1 -> Delay11/1
  Delay18/1 -> Delay12/1
  Delay19/1 -> Delay13/1
  Delay20/1 -> Delay14/1
  Delay21/1 -> Delay17/1, Delay15/1
  Delay22/1 -> Delay16/1
  Delay23/1 -> Delay21/1
  Data Type Conversion/1 -> Delay28/1, Delay27/1, Delay24/1  "u016"
  Delay24/1 -> 1-D Lookup Table/1
  Delay25/1 -> Delay18/1
  Delay26/1 -> Delay19/1
  Delay27/1 -> 1-D Lookup Table1/1
  Delay28/1 -> 1-D Lookup Table2/1
  Delay29/1 -> Delay20/1
  Delay30/1 -> Delay29/1

== system soc_dvbs2_fpga/DVBS2/DVBS2 TxRx/Channel/AWGN Generator/Unit Variance Gaussian Noise/logImplementation/log/RangeReconstruction ==
  y_e : Inport
  exp_e : Inport  Port=2
  Add1 : Sum  Inputs=-+  OutDataTypeStr=fixdt(0,31,24)
  Bit Shift : hdlsllib/Logic and Bit Operations/Bit Shift  mode=Shift Left Logical  N=1
  Constant : Constant  Value=log(2)  OutDataTypeStr=fixdt(1,33,32)  SampleTime=-1
  Delay{1..6} (6 alike) : Delay
  Product : Product  OutDataTypeStr=fixdt(1,35,28)
  e : Outport
  wires:
  Bit Shift/1 -> e/1
  Product/1 -> Delay4/1
  Add1/1 -> Delay6/1
  Constant/1 -> Delay2/1
  exp_e/1 -> Delay3/1
  y_e/1 -> Delay1/1
  Delay3/1 -> Product/1
  Delay1/1 -> Delay5/1
  Delay2/1 -> Product/2
  Delay5/1 -> Add1/1
  Delay4/1 -> Add1/2
  Delay6/1 -> Bit Shift/1

== system soc_dvbs2_fpga/DVBS2/DVBS2 TxRx/Channel/AWGN Generator/Unit Variance Gaussian Noise/logImplementation/log/RangeReduction ==
  note: Range of x_e=[1,2)
  x : Inport
  Add : Sum  OutDataTypeStr=fixdt(0,49,48)
  Constant : Constant  OutDataTypeStr=uint8  SampleTime=-1
  Delay : Delay
  Delay{1,3..7} (6 alike) : Delay  DelayLength=1
  Delay2 : Delay
  Shift Arithmetic3 : ArithShift  BitShiftNumberSource=Input port  BitShiftNumber=8  BitShiftDirection=Left
      settings: InputPortMap=u0,p1
  leadingZeroDetector : MATLAB Function  TreatAsAtomicUnit=on
  x_e : Outport
  exp_e : Outport  Port=2  VectorParamsAs1DForOutWhenUnconnected=off
  wires:
  Delay2/1 -> Delay5/1, Shift Arithmetic3/2
  leadingZeroDetector/1(exp_e) -> Delay2/1  "exp_e-1"
  Delay1/1 -> leadingZeroDetector/1(x)
  Add/1 -> Delay6/1
  Delay/1 -> Shift Arithmetic3/1
  Shift Arithmetic3/1 -> Delay4/1  "x_e"
  Constant/1 -> Add/2
  x/1 -> Delay3/1, Delay1/1
  Delay3/1 -> Delay/1
  Delay4/1 -> Add/1
  Delay5/1 -> Delay7/1
  Delay6/1 -> x_e/1
  Delay7/1 -> exp_e/1

== system soc_dvbs2_fpga/DVBS2/DVBS2 TxRx/DVB-S2 HDL Receiver/Demod Deinterleave and FECDecode/DVBS2 HDL Deinterleaver/RAM Address Generator/Generate and Add Read Base Address/Indicate End of Every ShortFrame Length Samples ==
  readAddr : Inport
  Compare To Constant : simulink/Logic and Bit Operations/Compare To Constant  relop===  const=ConfigRx.ShortFrameLen - 1  OutDataTypeStr=boolean
  Compare To Constant1 : simulink/Logic and Bit Operations/Compare To Constant  relop===  const=ConfigRx.ShortFrameLen*2 - 1  OutDataTypeStr=boolean
  Compare To Constant2 : simulink/Logic and Bit Operations/Compare To Constant  relop===  const=ConfigRx.ShortFrameLen*3 - 1  OutDataTypeStr=boolean
  Compare To Constant3 : simulink/Logic and Bit Operations/Compare To Constant  relop===  const=ConfigRx.ShortFrameLen*4 - 1  OutDataTypeStr=boolean
  Logical Operator1 : Logic  Operator=OR  Inputs=4  AllPortsSameDT=off  OutDataTypeStr=boolean
  endIndicate : Outport
  wires:
  Logical Operator1/1 -> endIndicate/1
  Compare To Constant/1 -> Logical Operator1/1
  Compare To Constant3/1 -> Logical Operator1/4
  Compare To Constant1/1 -> Logical Operator1/2
  Compare To Constant2/1 -> Logical Operator1/3
  readAddr/1 -> Compare To Constant3/1, Compare To Constant2/1, Compare To Constant/1, Compare To Constant1/1

== system soc_dvbs2_fpga/DVBS2/DVBS2 TxRx/DVB-S2 HDL Receiver/Demod Deinterleave and FECDecode/DVBS2 HDL Deinterleaver/RAM Address Generator/Generate and Add Read Base Address/No HDL Read Address Debug Scope ==
  note: Base Address Index:
      | Remains constant till the end of the frame.
      | changes by 1 after every short and by 4 after every normal frame
  note: This subsystem is a copy of
      | Wrap Address subsystem
      | in the RAM subsystem
  note: Offset Address :
      | Each ramp signal in the time scope indicates a column pickup.
      | 1,3,4,5 ramp signals in constant base address index indicates a frame demodulated from QPSK, 8 PSK, 16 APSK, 32 APSK symbols respectively.
      | The height of the ramps indicates a normal or a short frame
  note: For Deinterleaver :
  note: Connect these line to Time scope to visualize signals
  baseAddrIdx : Inport
  captureBaseAddrIdx : Inport  Port=2
  offsetAddr : Inport  Port=3
  basePlusOffsetAddr : Inport  Port=4
  Add1 : Sum  Inputs=+-|
  Delay1 : Delay
  Delay14 : Delay  DelayLength=4
  Terminator{,1..4} (5 alike) : Terminator
  Unit Delay Enabled Synchronous : hdlsllib/Discrete/Unit Delay Enabled Synchronous  InitialCondition=0.0  SampleTime=-1
  Wrap Address : Subsystem
  wires:
  Delay1/1 -> Unit Delay Enabled Synchronous/2
  Delay14/1 -> Unit Delay Enabled Synchronous/1
  basePlusOffsetAddr/1 -> Add1/1, Terminator2/1, Wrap Address/1(u)  "Actual Address = Base Address Index * 16200 + Offset Address"
  offsetAddr/1 -> Terminator/1  "Offset Address"
  Unit Delay Enabled Synchronous/1 -> Terminator1/1  "Base Address Index"
  Add1/1 -> Terminator4/1  "Actual Address - Wrapped Actual Address"
  captureBaseAddrIdx/1 -> Delay1/1
  Wrap Address/1(y) -> Add1/2, Terminator3/1  "Wrapped Actual Address"
  baseAddrIdx/1 -> Delay14/1

== system soc_dvbs2_fpga/DVBS2/DVBS2 TxRx/DVB-S2 HDL Receiver/Demod Deinterleave and FECDecode/DVBS2 HDL Deinterleaver/RAM Address Generator/Read Offset Address/Compute Read Offset Address ==
  curR : Inport
  maxC : Inport  Port=2
  curC : Inport  Port=3
  Add : Sum  OutDataTypeStr=Inherit: Same as first input
  Delay1 : Delay  DelayLength=1
  Delay2 : Delay
  Delay3 : Delay
  Delay4 : Delay  DelayLength=1
  Delay5 : Delay  DelayLength=1
  Delay8 : Delay
  Product : Product  OutDataTypeStr=fixdt('ufix17')
  addr : Outport
  wires:
  Delay5/1 -> addr/1
  Delay4/1 -> Add/2
  Delay1/1 -> Add/1
  curC/1 -> Delay3/1
  Delay8/1 -> Product/1
  Delay3/1 -> Delay4/1
  curR/1 -> Delay8/1
  maxC/1 -> Delay2/1
  Product/1 -> Delay1/1
  Delay2/1 -> Product/2
  Add/1 -> Delay5/1

== system soc_dvbs2_fpga/DVBS2/DVBS2 TxRx/DVB-S2 HDL Receiver/Demod Deinterleave and FECDecode/DVBS2 HDL Deinterleaver/RAM Address Generator/Read Offset Address/Generate Signal for End of Frame ==
  maxR : Inport
  maxC : Inport  Port=2
  Add : Sum  Inputs=+-  OutDataTypeStr=Inherit: Same as first input
  Compare To Constant : simulink/Logic and Bit Operations/Compare To Constant  relop=~=  const=0  OutDataTypeStr=boolean
  Constant : Constant  OutDataTypeStr=fixdt('ufix1')  SampleTime=Tsamp
  Constant1 : Constant  Value=0  OutDataTypeStr=fixdt('ufix1')  SampleTime=Tsamp
  Delay : Delay
  Delay1 : Delay
  Delay2 : Delay  DelayLength=1
  Delay4 : Delay  DelayLength=1
  Product : Product  OutDataTypeStr=Inherit: Same as first input
  Switch : Switch  Criteria=u2 > Threshold  SaturateOnIntegerOverflow=off  InputSameDT=off
  chkwrAddrEnd : Outport
  wires:
  Compare To Constant/1 -> Switch/2
  Constant1/1 -> Switch/3
  Switch/1 -> Add/2
  Delay2/1 -> Add/1, Compare To Constant/1
  maxR/1 -> Delay/1
  Constant/1 -> Switch/1
  Add/1 -> Delay4/1
  Delay1/1 -> Product/2
  Delay/1 -> Product/1
  Delay4/1 -> chkwrAddrEnd/1
  maxC/1 -> Delay1/1
  Product/1 -> Delay2/1

== system soc_dvbs2_fpga/DVBS2/DVBS2 TxRx/DVB-S2 HDL Receiver/Stream Recovery/BB Decoder/Extract Stream/Extract User Packet /Indicate SYNCD bit ==
  rst : Inport
  Distance : Inport  Port=2
  validIn : Inport  Port=3
  Constant1 : Constant  OutDataTypeStr=fixdt(0,1,0)  SampleTime=-1
  Constant2 : Constant  Value=0  OutDataTypeStr=fixdt(0,1,0)  SampleTime=-1
  HDL Counter1 : hdlsllib/Sources/HDL Counter  CountType=Free running  CountInit=0  CountStep=1  CountMax=25  CountFromType=Initial value  CountFrom=0  CountResetPort=on  CountLoadPort=off  CountEnbPort=on  CountDirPort=off  CountHitOutputPort=off  CountDataType=Unsigned  CountWordLen=16  CountFracLen=0  CountSampTime=1
  Logical Operator3 : Logic  AllPortsSameDT=off  OutDataTypeStr=boolean
  Relational Operator1 : RelationalOperator  Operator===  OutDataTypeStr=boolean  RndMeth=Simplest  InputSameDT=off
  Subtract1 : Sum  Inputs=+-  OutDataTypeStr=Inherit: Same as first input
  Switch : Switch  Criteria=u2 ~= 0  SaturateOnIntegerOverflow=off  InputSameDT=off
  trigger : Outport
  wires:
  rst/1 -> HDL Counter1/1
  Logical Operator3/1 -> trigger/1
  Switch/1 -> Subtract1/2
  validIn/1 -> HDL Counter1/2, Logical Operator3/2
  Distance/1 -> Subtract1/1, Switch/2
  Subtract1/1 -> Relational Operator1/1
  Relational Operator1/1 -> Logical Operator3/1
  Constant2/1 -> Switch/3
  Constant1/1 -> Switch/1
  HDL Counter1/1 -> Relational Operator1/2

== system soc_dvbs2_fpga/DVBS2/DVBS2 TxRx/DVB-S2 HDL Receiver/Synchronizer and PL Header Decoder/PL Header Recovery/PL Header Decoder/ML Decoder/Compute Euclidean Distance ==
  softBit : Inport
  Add : Sum  Inputs=+-+
  Add1 : Sum  Inputs=+++
  Constant : Constant  OutDataTypeStr=fixdt(0,1,0)  SampleTime=-1
  Data Type Duplicate : DataTypeDuplicate
  Data Type Conversion : DataTypeConversion  SaturateOnIntegerOverflow=off  RndMeth=Floor
  Delay{1..7} (7 alike) : Delay
  Divide by 2 : DataTypeConversion  OutDataTypeStr=fixdt(1,18,12)  ConvertRealWorld=Stored Integer (SI)  SaturateOnIntegerOverflow=off  RndMeth=Floor
  Product : Product  OutDataTypeStr=Inherit: Same as first input
  forBit0 : Outport
  forBit1 : Outport  Port=2
  wires:
  Data Type Conversion/1 -> forBit1/1, Data Type Duplicate/2
  Add1/1 -> forBit0/1, Data Type Duplicate/1
  Delay1/1 -> Product/1
  Delay6/1 -> Add1/2
  Delay3/1 -> Add1/3, Add/1
  Delay2/1 -> Product/2
  Product/1 -> Delay3/1
  Delay7/1 -> Add/2
  Delay4/1 -> Delay7/1
  Delay5/1 -> Delay6/1
  Divide by 2/1 -> Delay4/1, Delay5/1
  softBit/1 -> Delay1/1, Delay2/1, Divide by 2/1
  Add/1 -> Data Type Conversion/1
  Constant/1 -> Add1/1, Add/3

== system soc_dvbs2_fpga/DVBS2/DVBS2 TxRx/DVB-S2 HDL Receiver/Synchronizer and PL Header Decoder/PL Header Recovery/PL Header Decoder/ML Decoder/Euclidean Distance Sum Up ==
  Ed0 : Inport
  Ed1 : Inport  Port=2
  reset : Inport  Port=3
  CWswitch : Inport  Port=4  Partition=on  PartitionDimension=1  PartitionWidth=1  PartitionOffset=0
  validIn : Inport  Port=5
  Add : Sum  OutDataTypeStr=Inherit: Inherit via back propagation
  Data Type Duplicate : DataTypeDuplicate
  Delay{1..4} (4 alike) : Delay  DelayLength=1
  For Each : ForEach  DisableCoverage=on
  Switch : Switch  Criteria=u2 ~= 0  SaturateOnIntegerOverflow=off  InputSameDT=off
  Unit Delay Enabled Resettable Synchronous : hdlsllib/Discrete/Unit Delay Enabled Resettable Synchronous  InitialCondition=0.0  SampleTime=-1
  CwEdMetric : Outport  ConcatenationDimension=1
  wires:
  Delay4/1 -> CwEdMetric/1
  Delay2/1 -> Unit Delay Enabled Resettable Synchronous/3
  Delay1/1 -> Unit Delay Enabled Resettable Synchronous/2
  Delay3/1 -> Add/2, Data Type Duplicate/1
  reset/1 -> Delay2/1
  Add/1 -> Unit Delay Enabled Resettable Synchronous/1, Data Type Duplicate/2
  validIn/1 -> Delay1/1
  Unit Delay Enabled Resettable Synchronous/1 -> Delay4/1, Add/1
  Switch/1 -> Delay3/1
  Ed0/1 -> Switch/3
  Ed1/1 -> Switch/1
  CWswitch/1 -> Switch/2

== system soc_dvbs2_fpga/DVBS2/DVBS2 TxRx/DVB-S2 HDL Receiver/Synchronizer and PL Header Decoder/PL Header Recovery/PL Header Decoder/ML Decoder/Get Min Index ==
  dataIn : Inport
  validIn : Inport  Port=2
  Delay{1..6} (6 alike) : Delay  DelayLength=3
  For Each Subsystem : Subsystem  TreatAsAtomicUnit=on
  For Each Subsystem1 : Subsystem  TreatAsAtomicUnit=on
  For Each Subsystem2 : Subsystem  TreatAsAtomicUnit=on
  For Each Subsystem3 : Subsystem  TreatAsAtomicUnit=on
  For Each Subsystem4 : Subsystem  TreatAsAtomicUnit=on
  For Each Subsystem5 : Subsystem  TreatAsAtomicUnit=on
  indices : Constant  Value=(0:63).'  OutDataTypeStr=fixdt(0,6,0)  SampleTime=-1
  out : Outport
  validOut : Outport  Port=2
  wires:
  Delay6/1 -> validOut/1
  Delay5/1 -> Delay6/1
  Delay4/1 -> Delay5/1
  Delay2/1 -> Delay4/1
  Delay1/1 -> Delay2/1
  Delay3/1 -> Delay1/1
  For Each Subsystem5/1(idxOut) -> out/1
  For Each Subsystem4/2(idxOut) -> For Each Subsystem5/2(idxIn)
  For Each Subsystem4/1(ValueOut) -> For Each Subsystem5/1(valueIn)
  For Each Subsystem3/2(idxOut) -> For Each Subsystem4/2(idxIn)
  For Each Subsystem3/1(ValueOut) -> For Each Subsystem4/1(valueIn)
  For Each Subsystem2/2(idxOut) -> For Each Subsystem3/2(idxIn)
  For Each Subsystem2/1(ValueOut) -> For Each Subsystem3/1(valueIn)
  For Each Subsystem1/2(idxOut) -> For Each Subsystem2/2(idxIn)
  For Each Subsystem1/1(ValueOut) -> For Each Subsystem2/1(valueIn)
  validIn/1 -> Delay3/1
  For Each Subsystem/2(idxOut) -> For Each Subsystem1/2(idxIn)
  For Each Subsystem/1(ValueOut) -> For Each Subsystem1/1(valueIn)
  indices/1 -> For Each Subsystem/2(idxIn)
  dataIn/1 -> For Each Subsystem/1(valueIn)

== system soc_dvbs2_fpga/DVBS2/DVBS2 TxRx/DVB-S2 HDL Receiver/Synchronizer and PL Header Decoder/PL Header Recovery/PL Header Decoder/ML Decoder/Integer to Bit Convertor ==
  MS : Inport
  LS : Inport  Port=2
  For Each Subsystem : Subsystem  TreatAsAtomicUnit=on
  For Each Subsystem1 : Subsystem  TreatAsAtomicUnit=on
  For Each Subsystem2 : Subsystem  TreatAsAtomicUnit=on
  For Each Subsystem3 : Subsystem  TreatAsAtomicUnit=on
  For Each Subsystem4 : Subsystem  TreatAsAtomicUnit=on
  For Each Subsystem5 : Subsystem  TreatAsAtomicUnit=on
  For Each Subsystem6 : Subsystem  TreatAsAtomicUnit=on
  For Each Subsystem7 : Subsystem  TreatAsAtomicUnit=on
  Mux : Mux  Inputs=2
  Subsystem : Subsystem
  Subsystem1 : Subsystem
  Out1 : Outport
  wires:
  Mux/1 -> Out1/1
  LS/1 -> Subsystem1/1(u), Subsystem1/2(u1)
  For Each Subsystem4/1(Out1) -> For Each Subsystem5/1(In1)
  For Each Subsystem5/1(Out1) -> For Each Subsystem6/1(In1)
  For Each Subsystem6/1(Out1) -> For Each Subsystem7/1(In1)
  Subsystem1/1(Out1) -> For Each Subsystem4/1(In1)
  For Each Subsystem7/1(Out1) -> Mux/2
  For Each Subsystem3/1(Out1) -> Mux/1
  Subsystem/1(Out1) -> For Each Subsystem/1(In1)
  For Each Subsystem2/1(Out1) -> For Each Subsystem3/1(In1)
  For Each Subsystem1/1(Out1) -> For Each Subsystem2/1(In1)
  For Each Subsystem/1(Out1) -> For Each Subsystem1/1(In1)
  MS/1 -> Subsystem/2(u1), Subsystem/1(u)

== system soc_dvbs2_fpga/DVBS2/DVBS2 TxRx/DVB-S2 HDL Receiver/Synchronizer and PL Header Decoder/Time Frequency and Coarse Phase Synchronizer/Coarse Phase Synchronizer/Coarse Phase Corrector/Reciprocal ==
  dataIn : Inport
  Compare To Constant : simulink/Logic and Bit Operations/Compare To Constant  relop=<  const=0  OutDataTypeStr=boolean
  Data Type Conversion : DataTypeConversion  OutDataTypeStr=fixdt(1,WL,0)  ConvertRealWorld=Stored Integer (SI)  SaturateOnIntegerOverflow=off  RndMeth=Floor
  Data Type Conversion1 : DataTypeConversion  OutDataTypeStr=fixdt(0,LUTAddrWL,0)  ConvertRealWorld=Stored Integer (SI)  SaturateOnIntegerOverflow=off  RndMeth=Floor
  Data Type Conversion2 : DataTypeConversion  OutDataTypeStr=fixdt(0,WL-LUTAddrWL,0)  ConvertRealWorld=Stored Integer (SI)  SaturateOnIntegerOverflow=off  RndMeth=Floor
  Delay : Delay  DelayLength=1
  Delay1 : Delay  DelayLength=1
  Delay2 : Delay  DelayLength=1
  Extract Bits : simulink/Logic and Bit Operations/Extract Bits  bitsToExtract=Range ending with least significant bit  numBits=LUTAddrWL  bitIdxRange=[0 7]  outScalingMode=Treat bit field as an integer
  Function Impl : Subsystem
  dataOut : Outport
  wires:
  Data Type Conversion2/1 -> Function Impl/1(switch)
  Delay2/1 -> Data Type Conversion1/1
  Delay1/1 -> Data Type Conversion2/1
  Delay/1 -> Extract Bits/1, Compare To Constant/1
  Function Impl/1(functionValues) -> dataOut/1
  Data Type Conversion1/1 -> Function Impl/2(LUTAddr)
  Compare To Constant/1 -> Delay1/1
  Data Type Conversion/1 -> Delay/1
  Extract Bits/1 -> Delay2/1
  dataIn/1 -> Data Type Conversion/1
